simulink model "close_loop_tf2"  (R2017a)
settings: Solver=VariableStepAuto  StartTime=0.0  StopTime=20  RelTol=1e-3
libraries: simulink x2, dspsrcs4 x1
settings Model: Creator=ljxia_000  LastModifiedBy=ljxia

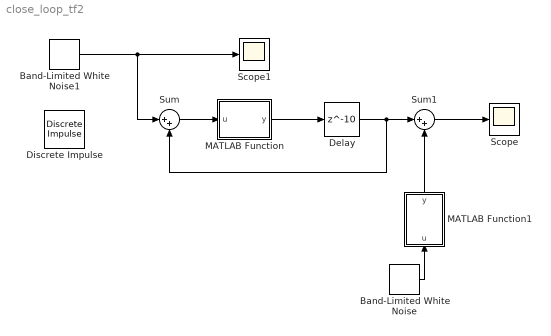
== system close_loop_tf2 ==
  Band-Limited White Noise : simulink/Sources/Band-Limited White Noise  Cov=[0.1]  Ts=0.1  seed=[23341]
  Band-Limited White Noise1 : simulink/Sources/Band-Limited White Noise  Cov=[0.1]  Ts=0.1  seed=[23331]
  Delay : Delay  DelayLength=10  InitialCondition=0
  Discrete Impulse : dspsrcs4/Discrete  Impulse  Delay=0  SampleTime=1  FrameSample=1  OutputFrames=off  dataType=double  isSigned=on  wordLen=16  udDataType=sfix(16)  fracBitsMode=Best precision  numFracBits=15  OutDataTypeStr=double  LastOutDataTypeStr=double
  MATLAB Function : MATLAB Function  TreatAsAtomicUnit=on
  MATLAB Function1 : MATLAB Function  TreatAsAtomicUnit=on
  Scope : Scope
  Scope1 : Scope
  Sum : Sum  Inputs=|++
  Sum1 : Sum  Inputs=|++
  wires:
  Sum/1 -> MATLAB Function/1(u)
  MATLAB Function/1(y) -> Delay/1
  Delay/1 -> Sum/2, Sum1/1
  Sum1/1 -> Scope/1
  Band-Limited White Noise/1 -> MATLAB Function1/1(u)
  MATLAB Function1/1(y) -> Sum1/2
  Band-Limited White Noise1/1 -> Sum/1, Scope1/1

== matlab function close_loop_tf2/MATLAB Function1 ==
  data: u input; y output
function y = fcn(u)
y = 0.71/(1-0.7*u^-1);

== matlab function close_loop_tf2/MATLAB Function ==
  data: u input; y output
function y = fcn(u)
Ts = 100;
y = 0.6*(1+Ts/50 -u^-1)/(1-u^-1);
